simulink model "MISSILE_CONTROL_SYSTEM"  (R2022b)
settings: Solver=VariableStepAuto  StartTime=0.0  StopTime=20  MaxStep=0.01  MinStep=0.001  RelTol=1e-6  AbsTol=1e-6
undefined symbols (not defined in the file): A, AC, B, BC, C, CC, K, k1, k2, kF
settings Model: Creator=siddi  LastModifiedBy=User
settings DebuggingCC: UnconnectedInputMsg=warning  UnconnectedOutputMsg=warning  UnconnectedLineMsg=warning
settings ModelReferenceCC: EnableRefExpFcnMdlSchedulingChecks=on
settings RTWCC: DLArmComputeVersion=19.05

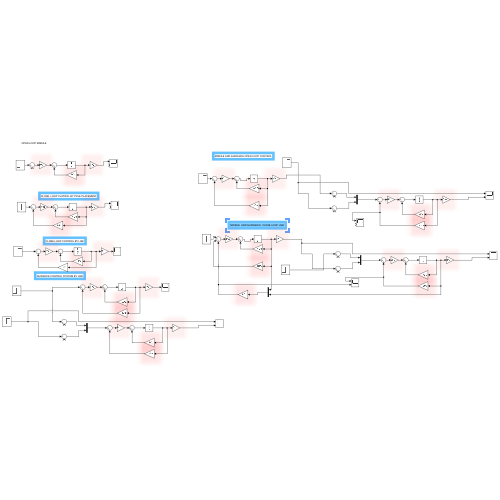
[thumbnail: Simulink's stored preview of the top-level diagram]
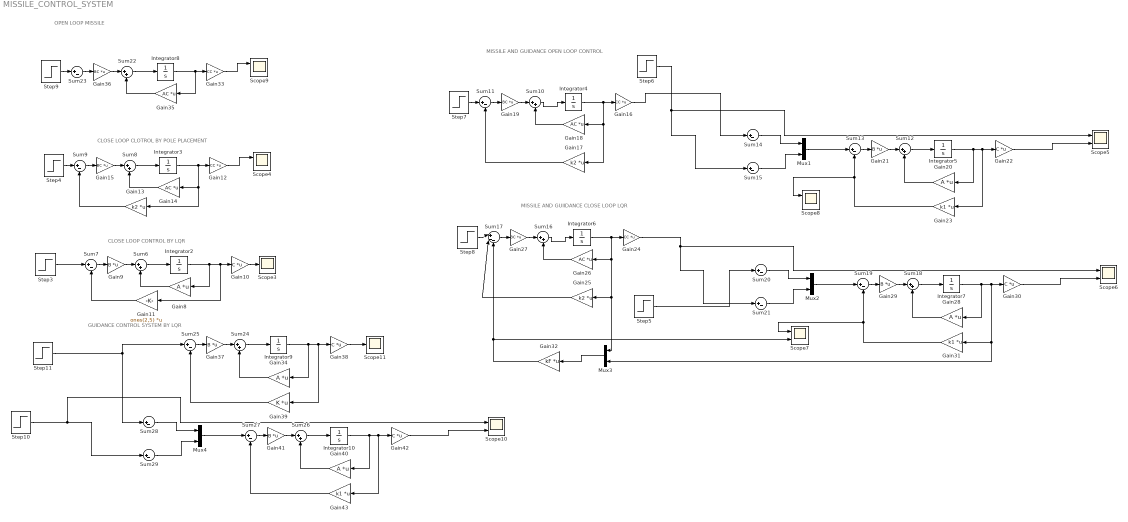
== system MISSILE_CONTROL_SYSTEM ==
  note: MISSILE AND GUIIDANCE CLOSE LOOP LQR
  note: MISSILE AND GUIDANCE OPEN LOOP CONTROL
  note: GUIDANCE CONTROL SYSTEM BY LQR
  note: CLOSE LOOP CONTROL BY LQR
  note: CLOSE LOOP CLOTROL BY POLE PLACEMENT
  note: OPEN LOOP MISSILE
  Gain{10,22,30,38,42} (5 alike) : Gain  Gain=C  Multiplication=Matrix(K*u)
  Gain11 : Gain  Gain=ones(2,5)  Multiplication=Matrix(K*u)
  Gain{12,16,24,33} (4 alike) : Gain  Gain=CC  Multiplication=Matrix(K*u)
  Gain13 : Gain  Gain=k2  Multiplication=Matrix(K*u)
  Gain{14,18,26,35} (4 alike) : Gain  Gain=AC  Multiplication=Matrix(K*u)
  Gain{15,19,27,36} (4 alike) : Gain  Gain=BC  Multiplication=Matrix(K*u)
  Gain17 : Gain  Gain=k2  Multiplication=Matrix(K*u)
  Gain{8,20,28,34,40} (5 alike) : Gain  Gain=A  Multiplication=Matrix(K*u)
  Gain{9,21,29,37,41} (5 alike) : Gain  Gain=B  Multiplication=Matrix(K*u)
  Gain23 : Gain  Gain=k1  Multiplication=Matrix(K*u)
  Gain25 : Gain  Gain=k2  Multiplication=Matrix(K*u)
  Gain31 : Gain  Gain=k1  Multiplication=Matrix(K*u)
  Gain32 : Gain  Gain=kF  Multiplication=Matrix(K*u)
  Gain39 : Gain  Gain=K  Multiplication=Matrix(K*u)
  Gain43 : Gain  Gain=k1  Multiplication=Matrix(K*u)
  Integrator{2..10} (9 alike) : Integrator
  Mux{1..4} (4 alike) : Mux  Inputs=2
  Scope{4..10} (7 alike) : Scope  NumInputPorts=2
  Scope11 : Scope
  Scope3 : Scope
  Step{3..11} (9 alike) : Step  SampleTime=0
  Sum{6,8,10,12,16,18,22,24,26} (9 alike) : Sum  Inputs=|++
  Sum{7,9,11,13..15,19..21,23,25,27..29} (14 alike) : Sum  Inputs=|+-
  Sum17 : Sum  Inputs=|+--
  wires:
  Gain16/1 -> Sum14/1
  Step5/1 -> Sum20/1
  Gain24/1 -> Sum21/1, Scope6/1
  Sum12/1 -> Integrator5/1
  Gain32/1 -> Scope7/2, Sum17/3
  Sum11/1 -> Gain19/1
  Gain19/1 -> Sum10/1
  Gain20/1 -> Sum12/2
  Sum16/1 -> Integrator6/1
  Gain29/1 -> Sum18/1
  Step8/1 -> Sum17/1
  Sum19/1 -> Gain29/1
  Gain31/1 -> Scope7/1, Sum19/2
  Gain17/1 -> Sum11/2
  Integrator7/1 -> Gain28/1, Mux3/2, Gain31/1, Gain30/1
  Gain18/1 -> Sum10/2
  Gain30/1 -> Scope6/2
  Sum20/1 -> Mux2/1
  Gain25/1 -> Sum17/2
  Gain26/1 -> Sum16/2
  Sum18/1 -> Integrator7/1
  Gain27/1 -> Sum16/1
  Mux2/1 -> Sum19/1
  Mux3/1 -> Gain32/1
  Integrator6/1 -> Mux3/1, Gain25/1, Gain26/1, Gain24/1
  Sum14/1 -> Mux1/1
  Mux1/1 -> Sum13/1
  Sum15/1 -> Mux1/2
  Gain22/1 -> Scope5/2
  Integrator5/1 -> Gain20/1, Gain23/1, Gain22/1
  Sum17/1 -> Gain27/1
  Sum21/1 -> Mux2/2
  Sum13/1 -> Gain21/1
  Integrator4/1 -> Gain17/1, Gain18/1, Gain16/1
  Step6/1 -> Sum15/1, Scope5/1
  Sum10/1 -> Integrator4/1
  Step7/1 -> Sum11/1
  Gain21/1 -> Sum12/1
  Gain23/1 -> Scope8/1, Sum13/2
  Gain28/1 -> Sum18/2
  Integrator9/1 -> Gain34/1, Gain39/1, Gain38/1
  Mux4/1 -> Sum27/1
  Step11/1 -> Sum28/1, Sum25/1
  Gain34/1 -> Sum24/2
  Gain39/1 -> Sum25/2
  Sum26/1 -> Integrator10/1
  Gain43/1 -> Sum27/2
  Sum29/1 -> Mux4/2
  Gain14/1 -> Sum8/2
  Gain41/1 -> Sum26/1
  Integrator3/1 -> Gain13/1, Gain14/1, Gain12/1
  Integrator10/1 -> Gain40/1, Gain43/1, Gain42/1
  Gain38/1 -> Scope11/1
  Gain15/1 -> Sum8/1
  Step9/1 -> Sum23/1
  Sum24/1 -> Integrator9/1
  Gain33/1 -> Scope9/1
  Integrator8/1 -> Gain35/1, Gain33/1
  Gain42/1 -> Scope10/2
  Gain36/1 -> Sum22/1
  Sum27/1 -> Gain41/1
  Gain35/1 -> Sum22/2
  Step10/1 -> Scope10/1, Sum29/1
  Sum22/1 -> Integrator8/1
  Sum8/1 -> Integrator3/1
  Gain10/1 -> Scope3/1
  Sum23/1 -> Gain36/1
  Sum7/1 -> Gain9/1
  Step3/1 -> Sum7/1
  Integrator2/1 -> Gain8/1, Gain11/1, Gain10/1
  Gain9/1 -> Sum6/1
  Gain11/1 -> Sum7/2
  Sum28/1 -> Mux4/1
  Gain13/1 -> Sum9/2
  Step4/1 -> Sum9/1
  Gain37/1 -> Sum24/1
  Sum6/1 -> Integrator2/1
  Sum9/1 -> Gain15/1
  Gain40/1 -> Sum26/2
  Sum25/1 -> Gain37/1
  Gain12/1 -> Scope4/1
  Gain8/1 -> Sum6/2
